simulink library "combinedHighLowFreqData_cl"  (R2018b)
settings: Solver=VariableStepAuto  StartTime=0.0  StopTime=10.0  RelTol=1e-3
undefined symbols (not defined in the file): flw, hFlw
libraries: highFreqFlowData_ul x1, lowFreqFlowData_ul x1
settings Model: Creator=jcreed2  LastModifiedBy=mcobb

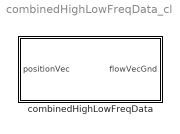
== system combinedHighLowFreqData_cl ==
  combinedHighLowFreqData : Subsystem  mask{flw=flw, hFlw=hFlw}
      mask prompts: flw "Low Frequency Flow Object"; hFlw "High Frequency Flow Object"

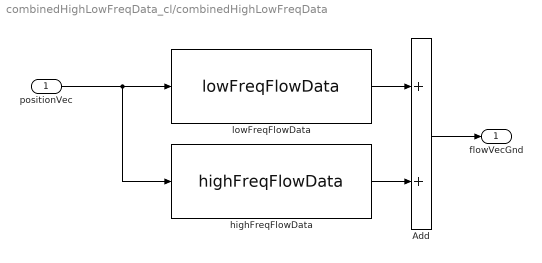
== system combinedHighLowFreqData_cl/combinedHighLowFreqData ==
  positionVec : Inport
  Add : Sum
  highFreqFlowData : highFreqFlowData_ul/highFreqFlowData  flw=flw  hFlw=hFlw
  lowFreqFlowData : lowFreqFlowData_ul/lowFreqFlowData  VariantControl=VSS_flowCalculation_constXYZT  flw=flw
  flowVecGnd : Outport
  wires:
  positionVec/1 -> highFreqFlowData/1, lowFreqFlowData/1
  lowFreqFlowData/1 -> Add/1
  highFreqFlowData/1 -> Add/2
  Add/1 -> flowVecGnd/1
